simulink model "PHIL_PLL"  (R2016a)
settings: Solver=FixedStepDiscrete  SolverMode=SingleTasking  StartTime=0.0  StopTime=1  FixedStep=2e-4  RelTol=1e-3
libraries: simulink x1, powerlib_meascontrol x1
settings Model: Creator=CoSES_HPC2  LastModifiedBy=CoSES_HPC2
settings DataIOCC: ReturnWorkspaceOutputs=on
settings DebuggingCC: RootOutportRequireBusObject=error  StrictBusMsg=ErrorOnBusTreatedAsVector  SFUnexpectedBacktrackingDiag=error  SFNoUnconditionalDefaultTransitionDiag=error
settings HardwareCC: ProdBitPerPointer=32  ProdLargestAtomicFloat=None  ProdWordSize=32  ProdHWDeviceType=Intel->x86/Pentium
settings SFSimCC: SimUseLocalCustomCode=on
settings RTWCC: SystemTargetFile=NIVeriStand.tlc  TemplateMakefile=NIVeriStand_vc.tmf  Description=NI Phar Lap Real-Time & Windows Targets  RTWUseLocalCustomCode=on
settings STFCustomTargetCC: MatFileLogging=on  SystemTargetFile=NIVeriStand.tlc
settings GRTTargetCC: ParMdlRefBuildCompliant=off  CompOptLevelCompliant=off  ConcurrentExecutionCompliant=off  GeneratePreprocessorConditionals=Use local settings  CombineOutputUpdateFcns=off  CPPClassGenCompliant=off  GRTInterface=on  UseToolchainInfoCompliant=off
settings ConfigComp: CovMetricSettings=dwe  CovHtmlReporting=off  CovSaveCumulativeToWorkspaceVar=off  CovSaveSingleToWorkspaceVar=off  CovExternalEMLEnable=on

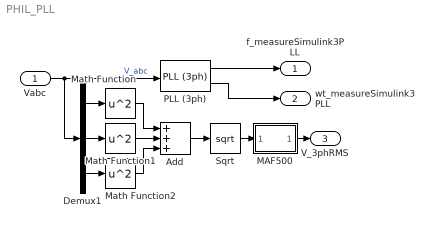
== system PHIL_PLL ==
  Vabc : Inport
  Add : Sum  Inputs=3
  Demux1 : Demux  Outputs=3
  MAF500 : Subsystem
  Math Function : Math  Operator=square  OutputSignalType=real  SaturateOnIntegerOverflow=on
  Math Function1 : Math  Operator=square  OutputSignalType=real  SaturateOnIntegerOverflow=on
  Math Function2 : Math  Operator=square  OutputSignalType=real  SaturateOnIntegerOverflow=on
  PLL (3ph) : powerlib_meascontrol/PLL/PLL (3ph)  Fmin=45  Par_Init=[0, 50]  ParK=[180, 3200, 1]  TcD=2e-4  MaxRateChangeFreq=12  FilterCutOffFreq=5  Ts=2e-4  AGC=on
  Sqrt : Sqrt  SaturateOnIntegerOverflow=on
  f_measureSimulink3PLL : Outport
  wt_measureSimulink3PLL : Outport  Port=2
  V_3phRMS : Outport  Port=3
  wires:
  Vabc/1 -> Demux1/1, PLL (3ph)/1  "V_abc"
  PLL (3ph)/1 -> f_measureSimulink3PLL/1
  PLL (3ph)/2 -> wt_measureSimulink3PLL/1
  Demux1/1 -> Math Function/1
  Demux1/2 -> Math Function1/1
  Demux1/3 -> Math Function2/1
  Math Function1/1 -> Add/2
  Math Function/1 -> Add/1
  Math Function2/1 -> Add/3
  Add/1 -> Sqrt/1
  Sqrt/1 -> MAF500/1(In1)
  MAF500/1(Out1) -> V_3phRMS/1

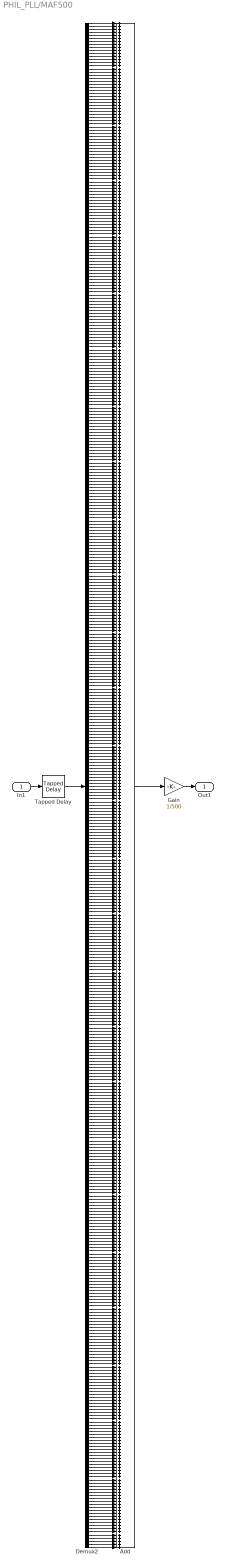
== system PHIL_PLL/MAF500 ==
  In1 : Inport
  Add : Sum  Inputs=500
  Demux2 : Demux  Outputs=500
  Gain : Gain  Gain=1/500
  Tapped Delay : simulink/Discrete/Tapped Delay  vinit=0  samptime=-1  NumDelays=500  DelayOrder=Newest  includeCurrent=off
  Out1 : Outport
  wires:
  Demux2/402 -> Add/402
  Demux2/418 -> Add/418
  Demux2/430 -> Add/430
  Demux2/423 -> Add/423
  Demux2/422 -> Add/422
  Demux2/442 -> Add/442
  Demux2/443 -> Add/443
  Demux2/345 -> Add/345
  Demux2/495 -> Add/495
  Demux2/397 -> Add/397
  Demux2/491 -> Add/491
  Demux2/344 -> Add/344
  Demux2/412 -> Add/412
  Demux2/398 -> Add/398
  Demux2/377 -> Add/377
  Demux2/487 -> Add/487
  Demux2/486 -> Add/486
  Demux2/439 -> Add/439
  Demux2/454 -> Add/454
  Demux2/413 -> Add/413
  Demux2/450 -> Add/450
  Demux2/160 -> Add/160
  Demux2/165 -> Add/165
  Demux2/302 -> Add/302
  Demux2/162 -> Add/162
  Demux2/210 -> Add/210
  Demux2/171 -> Add/171
  Demux2/161 -> Add/161
  Demux2/163 -> Add/163
  Demux2/166 -> Add/166
  Demux2/435 -> Add/435
  Demux2/335 -> Add/335
  Demux2/167 -> Add/167
  Demux2/164 -> Add/164
  Demux2/292 -> Add/292
  Demux2/313 -> Add/313
  Demux2/266 -> Add/266
  Demux2/334 -> Add/334
  Demux2/177 -> Add/177
  Demux2/168 -> Add/168
  Demux2/174 -> Add/174
  Demux2/169 -> Add/169
  Demux2/267 -> Add/267
  Demux2/170 -> Add/170
  Demux2/268 -> Add/268
  Demux2/287 -> Add/287
  Demux2/185 -> Add/185
  Demux2/173 -> Add/173
  Demux2/179 -> Add/179
  Demux2/471 -> Add/471
  Demux2/175 -> Add/175
  Demux2/176 -> Add/176
  Demux2/180 -> Add/180
  Demux2/172 -> Add/172
  Demux2/178 -> Add/178
  Demux2/182 -> Add/182
  Demux2/181 -> Add/181
  Demux2/298 -> Add/298
  Demux2/183 -> Add/183
  Demux2/294 -> Add/294
  Demux2/320 -> Add/320
  Demux2/277 -> Add/277
  Demux2/279 -> Add/279
  Demux2/278 -> Add/278
  Demux2/496 -> Add/496
  Demux2/484 -> Add/484
  Demux2/348 -> Add/348
  Demux2/308 -> Add/308
  Demux2/360 -> Add/360
  Demux2/297 -> Add/297
  Demux2/255 -> Add/255
  Demux2/201 -> Add/201
  Demux2/295 -> Add/295
  Demux2/205 -> Add/205
  Demux2/440 -> Add/440
  Demux2/356 -> Add/356
  Demux2/245 -> Add/245
  Demux2/209 -> Add/209
  Demux2/247 -> Add/247
  Demux2/211 -> Add/211
  Demux2/248 -> Add/248
  Demux2/219 -> Add/219
  Demux2/301 -> Add/301
  Demux2/490 -> Add/490
  Demux2/323 -> Add/323
  Demux2/322 -> Add/322
  Demux2/224 -> Add/224
  Demux2/433 -> Add/433
  Demux2/472 -> Add/472
  Demux2/260 -> Add/260
  Demux2/318 -> Add/318
  Demux2/225 -> Add/225
  Demux2/288 -> Add/288
  Demux2/238 -> Add/238
  Demux2/434 -> Add/434
  Demux2/239 -> Add/239
  Demux2/317 -> Add/317
  Demux2/231 -> Add/231
  Demux2/373 -> Add/373
  Demux2/311 -> Add/311
  Demux2/195 -> Add/195
  Demux2/374 -> Add/374
  Demux2/197 -> Add/197
  Demux2/259 -> Add/259
  Demux2/196 -> Add/196
  Demux2/381 -> Add/381
  Demux2/215 -> Add/215
  Demux2/124 -> Add/124
  Demux2/332 -> Add/332
  Demux2/150 -> Add/150
  Demux2/226 -> Add/226
  Demux2/125 -> Add/125
  Demux2/134 -> Add/134
  Demux2/214 -> Add/214
  Demux2/227 -> Add/227
  Demux2/499 -> Add/499
  Demux2/220 -> Add/220
  Demux2/391 -> Add/391
  Demux2/249 -> Add/249
  Demux2/140 -> Add/140
  Demux2/392 -> Add/392
  Demux2/251 -> Add/251
  Demux2/477 -> Add/477
  Demux2/478 -> Add/478
  Demux2/385 -> Add/385
  Demux2/283 -> Add/283
  Demux2/135 -> Add/135
  Demux2/250 -> Add/250
  Demux2/272 -> Add/272
  Demux2/274 -> Add/274
  Demux2/244 -> Add/244
  Demux2/232 -> Add/232
  Demux2/457 -> Add/457
  Demux2/414 -> Add/414
  Demux2/380 -> Add/380
  Demux2/262 -> Add/262
  Demux2/382 -> Add/382
  Demux2/273 -> Add/273
  Demux2/261 -> Add/261
  Demux2/141 -> Add/141
  Demux2/458 -> Add/458
  Demux2/256 -> Add/256
  Gain/1 -> Out1/1
  In1/1 -> Tapped Delay/1
  Demux2/24 -> Add/24
  Demux2/82 -> Add/82
  Demux2/265 -> Add/265
  Demux2/64 -> Add/64
  Demux2/28 -> Add/28
  Demux2/29 -> Add/29
  Demux2/35 -> Add/35
  Demux2/33 -> Add/33
  Demux2/12 -> Add/12
  Demux2/154 -> Add/154
  Demux2/152 -> Add/152
  Demux2/107 -> Add/107
  Demux2/41 -> Add/41
  Demux2/105 -> Add/105
  Demux2/22 -> Add/22
  Demux2/53 -> Add/53
  Demux2/34 -> Add/34
  Demux2/56 -> Add/56
  Demux2/40 -> Add/40
  Demux2/106 -> Add/106
  Demux2/151 -> Add/151
  Demux2/133 -> Add/133
  Demux2/108 -> Add/108
  Demux2/43 -> Add/43
  Demux2/481 -> Add/481
  Demux2/59 -> Add/59
  Demux2/110 -> Add/110
  Demux2/464 -> Add/464
  Demux2/159 -> Add/159
  Demux2/90 -> Add/90
  Demux2/91 -> Add/91
  Demux2/93 -> Add/93
  Demux2/97 -> Add/97
  Demux2/156 -> Add/156
  Demux2/88 -> Add/88
  Demux2/158 -> Add/158
  Demux2/87 -> Add/87
  Demux2/92 -> Add/92
  Demux2/415 -> Add/415
  Demux2/96 -> Add/96
  Demux2/155 -> Add/155
  Demux2/475 -> Add/475
  Demux2/233 -> Add/233
  Demux2/359 -> Add/359
  Demux2/17 -> Add/17
  Demux2/358 -> Add/358
  Demux2/463 -> Add/463
  Demux2/157 -> Add/157
  Demux2/204 -> Add/204
  Demux2/153 -> Add/153
  Demux2/234 -> Add/234
  Demux2/20 -> Add/20
  Demux2/49 -> Add/49
  Demux2/52 -> Add/52
  Demux2/404 -> Add/404
  Demux2/30 -> Add/30
  Demux2/46 -> Add/46
  Demux2/26 -> Add/26
  Demux2/221 -> Add/221
  Demux2/387 -> Add/387
  Demux2/476 -> Add/476
  Demux2/117 -> Add/117
  Demux2/459 -> Add/459
  Demux2/222 -> Add/222
  Demux2/116 -> Add/116
  Demux2/307 -> Add/307
  Demux2/115 -> Add/115
  Demux2/206 -> Add/206
  Demux2/198 -> Add/198
  Demux2/113 -> Add/113
  Demux2/386 -> Add/386
  Demux2/306 -> Add/306
  Demux2/482 -> Add/482
  Demux2/76 -> Add/76
  Demux2/86 -> Add/86
  Demux2/411 -> Add/411
  Demux2/77 -> Add/77
  Demux2/143 -> Add/143
  Demux2/142 -> Add/142
  Demux2/144 -> Add/144
  Demux2/94 -> Add/94
  Demux2/71 -> Add/71
  Demux2/254 -> Add/254
  Demux2/74 -> Add/74
  Demux2/85 -> Add/85
  Demux2/401 -> Add/401
  Demux2/89 -> Add/89
  Demux2/69 -> Add/69
  Demux2/10 -> Add/10
  Demux2/42 -> Add/42
  Demux2/405 -> Add/405
  Demux2/45 -> Add/45
  Demux2/99 -> Add/99
  Demux2/346 -> Add/346
  Demux2/39 -> Add/39
  Demux2/228 -> Add/228
  Demux2/4 -> Add/4
  Demux2/51 -> Add/51
  Demux2/95 -> Add/95
  Demux2/50 -> Add/50
  Demux2/7 -> Add/7
  Demux2/269 -> Add/269
  Demux2/339 -> Add/339
  Demux2/347 -> Add/347
  Demux2/399 -> Add/399
  Demux2/188 -> Add/188
  Demux2/427 -> Add/427
  Demux2/112 -> Add/112
  Demux2/469 -> Add/469
  Demux2/187 -> Add/187
  Demux2/109 -> Add/109
  Demux2/409 -> Add/409
  Demux2/2 -> Add/2
  Demux2/270 -> Add/270
  Demux2/47 -> Add/47
  Demux2/48 -> Add/48
  Demux2/44 -> Add/44
  Demux2/62 -> Add/62
  Demux2/3 -> Add/3
  Demux2/60 -> Add/60
  Demux2/365 -> Add/365
  Demux2/242 -> Add/242
  Demux2/18 -> Add/18
  Demux2/290 -> Add/290
  Demux2/54 -> Add/54
  Demux2/364 -> Add/364
  Tapped Delay/1 -> Demux2/1
  Demux2/500 -> Add/500
  Demux2/246 -> Add/246
  Demux2/57 -> Add/57
  Demux2/63 -> Add/63
  Demux2/55 -> Add/55
  Demux2/65 -> Add/65
  Demux2/5 -> Add/5
  Demux2/470 -> Add/470
  Demux2/9 -> Add/9
  Demux2/66 -> Add/66
  Demux2/11 -> Add/11
  Demux2/184 -> Add/184
  Demux2/15 -> Add/15
  Demux2/21 -> Add/21
  Demux2/6 -> Add/6
  Demux2/8 -> Add/8
  Demux2/1 -> Add/1
  Demux2/19 -> Add/19
  Demux2/16 -> Add/16
  Demux2/14 -> Add/14
  Demux2/217 -> Add/217
  Demux2/216 -> Add/216
  Demux2/58 -> Add/58
  Demux2/37 -> Add/37
  Demux2/38 -> Add/38
  Demux2/27 -> Add/27
  Demux2/31 -> Add/31
  Demux2/32 -> Add/32
  Demux2/67 -> Add/67
  Demux2/61 -> Add/61
  Demux2/128 -> Add/128
  Demux2/126 -> Add/126
  Demux2/36 -> Add/36
  Demux2/258 -> Add/258
  Demux2/70 -> Add/70
  Demux2/428 -> Add/428
  Demux2/78 -> Add/78
  Demux2/68 -> Add/68
  Demux2/127 -> Add/127
  Demux2/83 -> Add/83
  Demux2/75 -> Add/75
  Demux2/81 -> Add/81
  Demux2/240 -> Add/240
  Demux2/73 -> Add/73
  Demux2/80 -> Add/80
  Demux2/330 -> Add/330
  Demux2/72 -> Add/72
  Demux2/79 -> Add/79
  Demux2/84 -> Add/84
  Demux2/241 -> Add/241
  Demux2/431 -> Add/431
  Demux2/23 -> Add/23
  Demux2/25 -> Add/25
  Demux2/13 -> Add/13
  Demux2/282 -> Add/282
  Add/1 -> Gain/1
  Demux2/299 -> Add/299
  Demux2/451 -> Add/451
  Demux2/446 -> Add/446
  Demux2/379 -> Add/379
  Demux2/300 -> Add/300
  Demux2/453 -> Add/453
  Demux2/400 -> Add/400
  Demux2/456 -> Add/456
  Demux2/341 -> Add/341
  Demux2/417 -> Add/417
  Demux2/309 -> Add/309
  Demux2/367 -> Add/367
  Demux2/390 -> Add/390
  Demux2/426 -> Add/426
  Demux2/352 -> Add/352
  Demux2/328 -> Add/328
  Demux2/366 -> Add/366
  Demux2/305 -> Add/305
  Demux2/289 -> Add/289
  Demux2/378 -> Add/378
  Demux2/291 -> Add/291
  Demux2/455 -> Add/455
  Demux2/383 -> Add/383
  Demux2/384 -> Add/384
  Demux2/280 -> Add/280
  Demux2/285 -> Add/285
  Demux2/319 -> Add/319
  Demux2/479 -> Add/479
  Demux2/395 -> Add/395
  Demux2/424 -> Add/424
  Demux2/394 -> Add/394
  Demux2/494 -> Add/494
  Demux2/396 -> Add/396
  Demux2/485 -> Add/485
  Demux2/296 -> Add/296
  Demux2/293 -> Add/293
  Demux2/350 -> Add/350
  Demux2/340 -> Add/340
  Demux2/337 -> Add/337
  Demux2/361 -> Add/361
  Demux2/349 -> Add/349
  Demux2/329 -> Add/329
  Demux2/447 -> Add/447
  Demux2/448 -> Add/448
  Demux2/321 -> Add/321
  Demux2/357 -> Add/357
  Demux2/315 -> Add/315
  Demux2/444 -> Add/444
  Demux2/303 -> Add/303
  Demux2/363 -> Add/363
  Demux2/372 -> Add/372
  Demux2/316 -> Add/316
  Demux2/371 -> Add/371
  Demux2/362 -> Add/362
  Demux2/441 -> Add/441
  Demux2/312 -> Add/312
  Demux2/375 -> Add/375
  Demux2/286 -> Add/286
  Demux2/425 -> Add/425
  Demux2/314 -> Add/314
  Demux2/284 -> Add/284
  Demux2/324 -> Add/324
  Demux2/376 -> Add/376
  Demux2/310 -> Add/310
  Demux2/449 -> Add/449
  Demux2/304 -> Add/304
  Demux2/421 -> Add/421
  Demux2/331 -> Add/331
  Demux2/281 -> Add/281
  Demux2/416 -> Add/416
  Demux2/445 -> Add/445
  Demux2/480 -> Add/480
  Demux2/271 -> Add/271
  Demux2/333 -> Add/333
  Demux2/276 -> Add/276
  Demux2/275 -> Add/275
  Demux2/436 -> Add/436
  Demux2/393 -> Add/393
  Demux2/452 -> Add/452
  Demux2/488 -> Add/488
  Demux2/199 -> Add/199
  Demux2/408 -> Add/408
  Demux2/189 -> Add/189
  Demux2/186 -> Add/186
  Demux2/149 -> Add/149
  Demux2/213 -> Add/213
  Demux2/139 -> Add/139
  Demux2/203 -> Add/203
  Demux2/194 -> Add/194
  Demux2/489 -> Add/489
  Demux2/137 -> Add/137
  Demux2/138 -> Add/138
  Demux2/336 -> Add/336
  Demux2/474 -> Add/474
  Demux2/212 -> Add/212
  Demux2/193 -> Add/193
  Demux2/118 -> Add/118
  Demux2/119 -> Add/119
  Demux2/473 -> Add/473
  Demux2/497 -> Add/497
  Demux2/420 -> Add/420
  Demux2/121 -> Add/121
  Demux2/406 -> Add/406
  Demux2/419 -> Add/419
  Demux2/123 -> Add/123
  Demux2/122 -> Add/122
  Demux2/403 -> Add/403
  Demux2/498 -> Add/498
  Demux2/207 -> Add/207
  Demux2/462 -> Add/462
  Demux2/131 -> Add/131
  Demux2/468 -> Add/468
  Demux2/147 -> Add/147
  Demux2/132 -> Add/132
  Demux2/148 -> Add/148
  Demux2/192 -> Add/192
  Demux2/191 -> Add/191
  Demux2/130 -> Add/130
  Demux2/342 -> Add/342
  Demux2/129 -> Add/129
  Demux2/343 -> Add/343
  Demux2/111 -> Add/111
  Demux2/389 -> Add/389
  Demux2/257 -> Add/257
  Demux2/465 -> Add/465
  Demux2/388 -> Add/388
  Demux2/354 -> Add/354
  Demux2/467 -> Add/467
  Demux2/483 -> Add/483
  Demux2/326 -> Add/326
  Demux2/466 -> Add/466
  Demux2/438 -> Add/438
  Demux2/437 -> Add/437
  Demux2/120 -> Add/120
  Demux2/202 -> Add/202
  Demux2/208 -> Add/208
  Demux2/136 -> Add/136
  Demux2/429 -> Add/429
  Demux2/229 -> Add/229
  Demux2/432 -> Add/432
  Demux2/243 -> Add/243
  Demux2/230 -> Add/230
  Demux2/410 -> Add/410
  Demux2/351 -> Add/351
  Demux2/146 -> Add/146
  Demux2/223 -> Add/223
  Demux2/325 -> Add/325
  Demux2/460 -> Add/460
  Demux2/327 -> Add/327
  Demux2/145 -> Add/145
  Demux2/218 -> Add/218
  Demux2/237 -> Add/237
  Demux2/264 -> Add/264
  Demux2/235 -> Add/235
  Demux2/338 -> Add/338
  Demux2/461 -> Add/461
  Demux2/114 -> Add/114
  Demux2/368 -> Add/368
  Demux2/263 -> Add/263
  Demux2/493 -> Add/493
  Demux2/253 -> Add/253
  Demux2/353 -> Add/353
  Demux2/407 -> Add/407
  Demux2/369 -> Add/369
  Demux2/252 -> Add/252
  Demux2/236 -> Add/236
  Demux2/102 -> Add/102
  Demux2/100 -> Add/100
  Demux2/98 -> Add/98
  Demux2/370 -> Add/370
  Demux2/103 -> Add/103
  Demux2/200 -> Add/200
  Demux2/355 -> Add/355
  Demux2/492 -> Add/492
  Demux2/101 -> Add/101
  Demux2/104 -> Add/104
  Demux2/190 -> Add/190
